simulink model "Exercise"  (R2018a)
settings: Solver=VariableStepAuto  StartTime=0.0  StopTime=inf  RelTol=1e-3
undefined symbols (not defined in the file): Rec, SDTV
libraries: dspvision x1, visionconversions x1, visionanalysis x1
settings Model: EnablePacing=on  Creator=놀러와마이홈  LastModifiedBy=놀러와마이홈

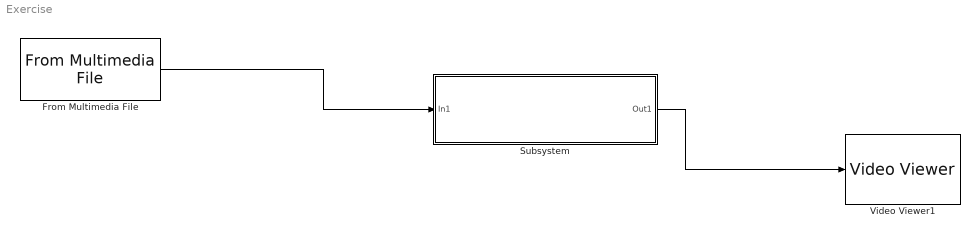
== system Exercise ==
  From Multimedia File : dspvision/From Multimedia File  inputFilename=C:\Users\놀러와마이홈\Documents\MATLAB\Lane Detection Test Video 01.mp4  loop=on  numPlays=inf  outputStreams=Video only  videoDataType=single  audioDataType=int16  inheritSampleTime=on  userDefinedSampleTime=1/30  noAudioOutput=off  isIntensityVideo=off  fourcc=RGB  colorVideoFormat=One multidimensional signal  outputEOF=off  dataOrg=Column-major  audioFrameSize=1024  computeAudioFrameSize=off  outSamplingMode=Sample based
      settings: SourceProductBaseCode=VP
  Subsystem : Subsystem  TreatAsAtomicUnit=on
  Video Viewer1 : VideoViewer  FigPos=[721.666666666667 576.666666666667 526 388.666666666667]
  wires:
  From Multimedia File/1 -> Subsystem/1(In1)
  Subsystem/1(Out1) -> Video Viewer1/1

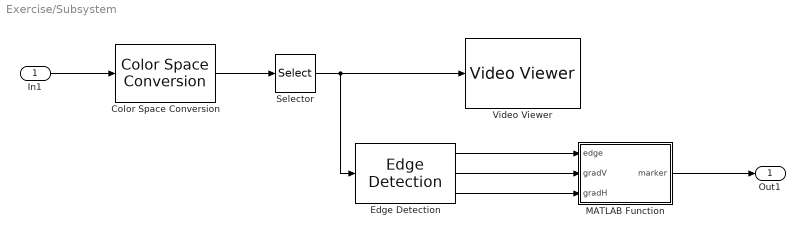
== system Exercise/Subsystem ==
  In1 : Inport
  Color Space Conversion : visionconversions/Color Space  Conversion  conversion=Obsolete  conversionActive=R'G'B' to intensity  wp_str=D65  rec=Rec. 601 (SDTV)  sys=1125/60/2:1  imagePorts=One multidimensional signal
      settings: SourceProductName=Computer Vision System Toolbox
  Edge Detection : visionanalysis/Edge Detection  method=Sobel  outputType=Binary image and gradient components  userDefinedThreshold=off  thresholdSource=Input port  threshold=20  thresholdTuning=4  edgeThinning=on  threshold_canny=[0.25 0.60]  autoPercent=70  sigma=1  roundingMode=Floor  overflowMode=off  prodOutputMode=Binary point scaling  prodOutputWordLength=32  prodOutputFracLength=8  prodOutputSlope=2^-8  accumSlope=2^-8  outputSlope=2^-4
      settings: SourceProductName=Computer Vision System Toolbox  SourceProductBaseCode=VP
  MATLAB Function : MATLAB Function  TreatAsAtomicUnit=on
  Selector : Selector  NumberOfDimensions=2  InputPortWidth=3  IndexOptions=Starting index (dialog),Starting index (dialog)  Indices=401,1  OutputSizes=320,1280
  Video Viewer : VideoViewer  FigPos=[185 576.666666666667 526 388.666666666667]
  Out1 : Outport
  wires:
  Edge Detection/2 -> MATLAB Function/2(gradV)
  In1/1 -> Color Space Conversion/1
  Edge Detection/1 -> MATLAB Function/1(edge)
  Edge Detection/3 -> MATLAB Function/3(gradH)
  Color Space Conversion/1 -> Selector/1
  Selector/1 -> Edge Detection/1, Video Viewer/1
  MATLAB Function/1(marker) -> Out1/1

== matlab function Exercise/Subsystem/MATLAB Function ==
  data: edge input; marker output; gradV input; gradH input
function marker = fcn(edge, gradV, gradH)

marker = zeros(size(edge),'logical');
for i=1:320
    for j=1:1280
        if edge(i,j)==false
            continue;
        end
        ang=atan2d(gradV(i,j),gradH(i,j));
        
        if abs(ang)<20||abs(ang)>180
            continue;
        end
        marker(i,j)=true;
    end
end
